simulink model "Quadcopter"  (R2024b)
settings: Solver=VariableStepAuto  StartTime=0.0  StopTime=1000  FixedStep=0.0001  RelTol=1e-3
values from neighbouring files (symbols this model uses):
  f = fn{i}    [LandingAnalysis.m]    (also in PerformanceAnalysis.m = @(a) obj.lift_residual(alt,V,M,rho,L_target,a,throttle); TakeoffAnalysis.m)
undefined symbols (not defined in the file or in its folder): Earth, WGS84
libraries: slpidlib x5, simulink_extras x2, aerolibfltsims x2, instrumentlib x2, shared6dof x1, vrlib x1, aerolibtransform2 x1, aerolibanimutils x1
settings Model: Creator=naman  LastModifiedBy=naman

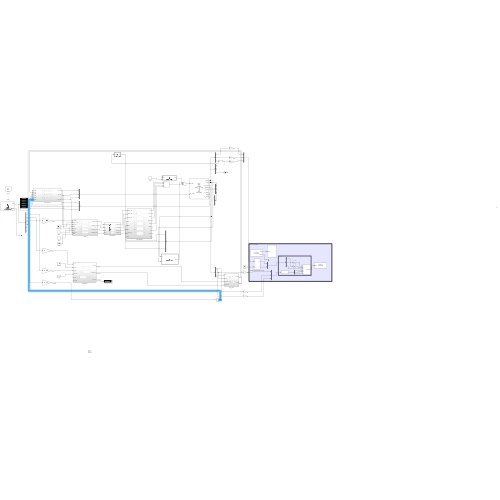
[thumbnail: Simulink's stored preview of the top-level diagram]
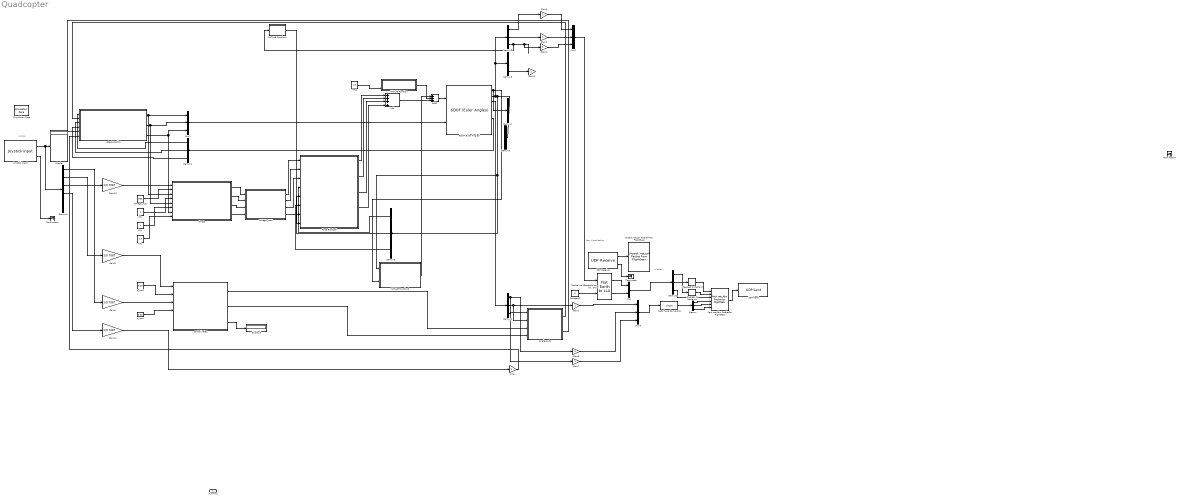
== system Quadcopter ==
  note: proiler
  note: Inertial
  note: New Visualization
  6DOF (Euler Angles) : shared6dof/6DOF (Euler Angles)  units=Metric (MKS)  mtype=Fixed  rep=Euler Angles  xme_0=[0;0;0]  Vm_0=[0;0;0]  eul_0=[0;0;0]  pm_0=[0;0;0]  mass_0=1.5  mass_e=0.5  mass_f=2.0  inertia=[0.06 0 0;0 0.06 0;0 0 0.10]  inertia_e=eye(3)  inertia_f=2*eye(3)  k_quat=1.0  vre_flag=on  abi_flag=off  aMode=0  xme_statename=''  Vm_statename=''  eul_statename=''  quat_statename=''  pm_statename=''  mass_statename=''
  Add : Sum  Inputs=++++
  Add2 : Sum  Inputs=+++
  Constant2 : Constant  Value=0
  Data Type Conversion : DataTypeConversion  OutDataTypeStr=single  SaturateOnIntegerOverflow=off  RndMeth=Floor
  Degrees to Radians : simulink_extras/Transformations/Degrees to Radians
  Degrees to Radians1 : simulink_extras/Transformations/Degrees to Radians
  Demux{,1..8} (9 alike) : Demux  Outputs=3
  Demux9 : Demux  Outputs=6
  Display : Display
  Display1 : Display
  Force Blockset : Subsystem
  Gain{1..4,6..7} (6 alike) : Gain
  Gain{8..11} (4 alike) : Gain  Gain=1/0.7087
  Gain5 : Gain  Gain=-1
  Joystick Input : vrlib/Joystick Input  joyid=1  adjustports=on  forcefeed=off
  MATLAB Function : MATLAB Function  TreatAsAtomicUnit=on
  MATLAB Function1 : MATLAB Function  TreatAsAtomicUnit=on
  MATLAB Function3 : MATLAB Function  TreatAsAtomicUnit=on
  Mux : Mux  Inputs=2
  Mux1 : Mux  Inputs=3
  Mux2 : Mux  Inputs=3
  Mux3 : Mux  Inputs=3
  Omega_max : Constant  Value=950
  Omega_rotor : Subsystem
  Omga : Subsystem
  Pack net_fdm Packet for FlightGear : aerolibfltsims/Pack net_fdm Packet for FlightGear  FlightGearVersion=v2019.1  ShowPositionAttitudeInputs=on  ShowVelocityAccelerationInputs=off  ShowControlSurfacePositionInputs=off  ShowEngineFuelInputs=off  ShowLandingGearInputs=off  ShowEnvironmentInputs=off  SampleTime=-1  packetVersion=24
  "Position to [Geodetic lat, lon, alti]" : aerolibtransform2/Flat Earth to LLA  units=Metric (MKS)  ptype=Earth (WGS84)  F=1/298.257223563  R=6378137  refPosPort=off  LL0=[37.210265015306916, -80.41446644179189]  psi=0
  Simulation Pace : aerolibanimutils/Simulation Pace  SimulationPace=1  SleepMode=Auto  OutputPaceError=off  SampleTime=1/30
  Terminator : Terminator
  Terminator1 : Terminator
  Terminator4 : Terminator
  UDP Receive : instrumentlib/UDP Receive  LocalAddress=127.0.0.1  LocalPort=50001  EnablePortSharing=off  Host=localhost  Port=65343  GetLatestData=on  DataSize=[ 1, 744 ]  DataType=uint8  ASCIIFormatting=%f,  Terminator=LF  CustomTerminator=10  ByteOrder=little-endian  EnableBlockingMode=off  Timeout=10  SampleTime=0.2  SimulateUsing=Interpreted execution
  UDP Send : instrumentlib/UDP Send  Host=localhost  Port=50000  LocalAddress=127.0.0.1  LocalPort=-1  EnablePortSharing=on  OutputDatagramPacketSize=4096  ByteOrder=big-endian  EnableBlockingMode=on  SimulateUsing=Interpreted execution
  Unpack net_ctrl Packet from FlightGear : aerolibfltsims/Unpack net_ctrl Packet from FlightGear  FlightGearVersion=v2019.1  ShowControlSurfacePositionOutputs=off  ShowEngineFuelOutputs=off  ShowLandingGearOutputs=off  ShowAvionicOutputs=off  ShowEnvironmentOutputs=off  SampleTime=-1  packetVersion=27
  angle_auto : Subsystem
  controll rates : Subsystem
  kMx : Constant  Value=4
  kMy : Constant  Value=4
  kMz : Constant  Value=1.5
  mass : Constant  Value=1.5
  p_max : Constant  Value=0.35
  q_max : Constant  Value=0.35
  r_max : Gain
  rate_Autopilot : Subsystem
  dummy2 : Outport
  wires:
  Demux/2 -> Pack net_fdm Packet for FlightGear/5
  Gain10/1 -> Omga/1(u_throttle)  "throttle"
  rate_Autopilot/1(Mx_cmd) -> Omga/3(Mx_cmd), Mux2/1
  kMz/1 -> Omga/8(kMz)
  Demux1/1 -> Degrees to Radians1/1
  Gain2/1 -> Mux1/2  "theta"
  Degrees to Radians1/1 -> Pack net_fdm Packet for FlightGear/2
  Degrees to Radians/1 -> Pack net_fdm Packet for FlightGear/1
  Demux/1 -> Pack net_fdm Packet for FlightGear/4
  controll rates/1(phi_cmd) -> angle_auto/3(phi_cmd)  "phi_cmd"
  Demux1/3 -> Pack net_fdm Packet for FlightGear/3
  Demux1/2 -> Degrees to Radians/1
  Data Type Conversion/1 -> Demux/1
  Omega_rotor/1(omega_FR) -> Force Blockset/1(Omega_FR)
  Demux/3 -> Pack net_fdm Packet for FlightGear/6
  Demux8/3 -> Force Blockset/6(psi)
  mass/1 -> MATLAB Function/3(m)
  UDP Receive/1 -> Unpack net_ctrl Packet from FlightGear/1
  rate_Autopilot/3(Mz_cmd) -> Omga/7(Mz_cmd), Mux2/3
  Demux9/2 -> Gain9/1  "roll"
  UDP Receive/2 -> Terminator/1
  Demux8/2 -> Force Blockset/5(theta)
  "Position to [Geodetic lat, lon, alti]"/1 -> Mux/1
  "Position to [Geodetic lat, lon, alti]"/2 -> Mux/2
  controll rates/3(psi_cmd) -> Display1/1  "psi_cmd"
  Omega_rotor/3(omega_RL) -> Force Blockset/3(Omega_RL)
  Joystick Input/1 -> Display/1, Demux9/1
  Joystick Input/2 -> Terminator1/1
  Demux9/1 -> Gain8/1
  q_max/1 -> controll rates/4(theta_max)
  Demux9/3 -> Gain10/1  "throttle"
  Demux8/1 -> Force Blockset/4(phi)
  Demux9/4 -> Gain11/1  "YAW"
  Force Blockset/5(Rrad) -> Add/3
  rate_Autopilot/2(My_cmd) -> Omga/5(My_cmd), Mux2/2
  Demux4/2 -> rate_Autopilot/3(q_6dof)
  Omega_max/1 -> Omga/2(Omega_max)
  Demux4/1 -> rate_Autopilot/1(p_6dof)
  kMx/1 -> Omga/4(kMx)
  kMy/1 -> Omga/6(kMy)
  Gain9/1 -> controll rates/1(u_roll)  "roll"
  p_max/1 -> controll rates/2(phi_max)
  Gain8/1 -> controll rates/3(u_pitch)  "pitch"
  Add/1 -> Add2/3
  Gain11/1 -> r_max/1  "u_yawYAW"
  Force Blockset/1(Front) -> Add/1
  MATLAB Function1/1(rho) -> Force Blockset/8(rho)
  Demux4/3 -> rate_Autopilot/4(r_6dof)
  Mux2/1 -> 6DOF (Euler Angles)/2
  Omga/1(Omega_base) -> Omega_rotor/1(Omega_base)
  Omga/2(dOmega_roll) -> Omega_rotor/2(dOr)
  Omga/3(dOmega_pitch) -> Omega_rotor/3(dOp)
  Omega_rotor/2(omega_RR) -> Force Blockset/2(Omega_RR)
  Omga/4(dOmega_yaw) -> Omega_rotor/4(dOy)
  controll rates/2(theta_cmd) -> angle_auto/4(theat_cmd)  "theta_cmd"
  Omega_rotor/4(omega_FL) -> Force Blockset/7(Omega_FL)
  Force Blockset/3(Right) -> Add/2
  Force Blockset/7(left) -> Add/4
  MATLAB Function/1(Fg_b) -> Add2/2
  MATLAB Function3/1(Fgnd_n) -> Add2/1
  Add2/1 -> 6DOF (Euler Angles)/1
  6DOF (Euler Angles)/1 -> Demux7/1, MATLAB Function3/2(Ve)
  6DOF (Euler Angles)/2 -> Demux8/1, MATLAB Function3/1(Xe), Demux6/1, Demux5/1, Demux2/1
  6DOF (Euler Angles)/3 -> Demux3/1
  6DOF (Euler Angles)/6 -> Demux4/1
  Demux2/1 -> Gain3/1
  Demux2/2 -> Gain2/1
  Demux2/3 -> Gain4/1, MATLAB Function1/1(Z_ned)  "z axis"
  Demux5/3 -> Gain5/1
  Demux3/1 -> Gain6/1, angle_auto/1(phi)  "phi"
  Demux3/2 -> Gain1/1, angle_auto/2(theta)  "theta"
  Demux3/3 -> Gain7/1  "psi"
  Gain3/1 -> Mux1/1  "phi"
  Gain4/1 -> Mux1/3  "psi"
  angle_auto/1(p_cmd) -> rate_Autopilot/2(p_cmd)  "p_cmd"
  angle_auto/2(q_cmd) -> rate_Autopilot/5(q_cmd)  "q_cmd"
  Pack net_fdm Packet for FlightGear/1 -> UDP Send/1
  Mux/1 -> Demux1/1
  Mux3/1 -> Data Type Conversion/1
  Mux1/1 -> "Position to [Geodetic lat, lon, alti]"/1
  Constant2/1 -> "Position to [Geodetic lat, lon, alti]"/2
  Gain1/1 -> Mux3/1  "theta"
  Gain6/1 -> Mux3/2  "phi"
  Gain7/1 -> Mux3/3  "psi"
  r_max/1 -> rate_Autopilot/6(r_cmd)  "r_cmd"

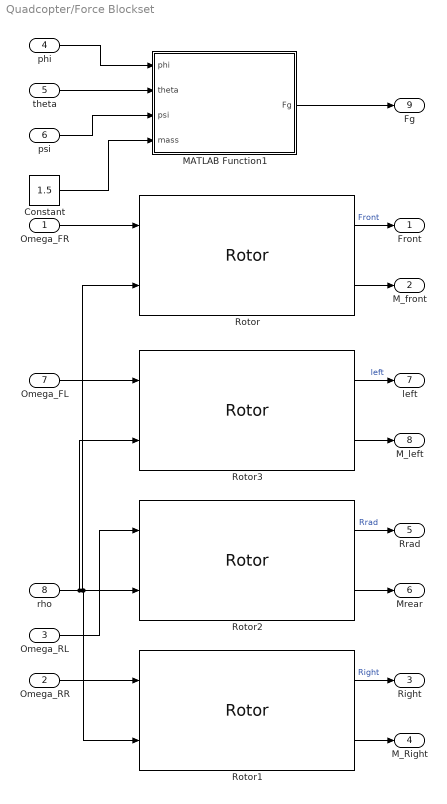
== system Quadcopter/Force Blockset ==
  Omega_FR : Inport
  Omega_RR : Inport  Port=2
  Omega_RL : Inport  Port=3
  phi : Inport  Port=4
  theta : Inport  Port=5
  psi : Inport  Port=6
  Omega_FL : Inport  Port=7
  rho : Inport  Port=8
  Constant : Constant  Value=1.5
  MATLAB Function1 : MATLAB Function  TreatAsAtomicUnit=on
  Rotor{,1..3} (4 alike) : Rotor  radius=0.127
  Front : Outport
  M_front : Outport  Port=2
  Right : Outport  Port=3
  M_Right : Outport  Port=4
  Rrad : Outport  Port=5
  Mrear : Outport  Port=6
  left : Outport  Port=7
  M_left : Outport  Port=8
  Fg : Outport  Port=9
  wires:
  phi/1 -> MATLAB Function1/1(phi)
  Omega_FL/1 -> Rotor3/1
  Omega_RL/1 -> Rotor2/1
  rho/1 -> Rotor1/2, Rotor2/2, Rotor/2, Rotor3/2
  theta/1 -> MATLAB Function1/2(theta)
  Omega_FR/1 -> Rotor/1
  Omega_RR/1 -> Rotor1/1
  psi/1 -> MATLAB Function1/3(psi)
  Constant/1 -> MATLAB Function1/4(mass)
  MATLAB Function1/1(Fg) -> Fg/1
  Rotor3/2 -> M_left/1
  Rotor/1 -> Front/1  "Front"
  Rotor/2 -> M_front/1
  Rotor3/1 -> left/1  "left"
  Rotor2/1 -> Rrad/1  "Rrad"
  Rotor2/2 -> Mrear/1
  Rotor1/1 -> Right/1  "Right"
  Rotor1/2 -> M_Right/1

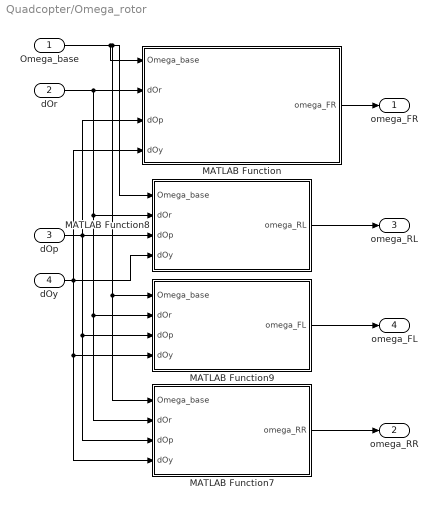
== system Quadcopter/Omega_rotor ==
  Omega_base : Inport
  dOr : Inport  Port=2
  dOp : Inport  Port=3
  dOy : Inport  Port=4
  MATLAB Function : MATLAB Function  TreatAsAtomicUnit=on
  MATLAB Function7 : MATLAB Function  TreatAsAtomicUnit=on
  MATLAB Function8 : MATLAB Function  TreatAsAtomicUnit=on
  MATLAB Function9 : MATLAB Function  TreatAsAtomicUnit=on
  omega_FR : Outport
  omega_RR : Outport  Port=2
  omega_RL : Outport  Port=3
  omega_FL : Outport  Port=4
  wires:
  MATLAB Function7/1(omega_RR) -> omega_RR/1
  MATLAB Function/1(omega_FR) -> omega_FR/1
  Omega_base/1 -> MATLAB Function9/1(Omega_base), MATLAB Function7/1(Omega_base), MATLAB Function8/1(Omega_base), MATLAB Function/1(Omega_base)
  dOy/1 -> MATLAB Function9/4(dOy), MATLAB Function7/4(dOy), MATLAB Function8/4(dOy), MATLAB Function/4(dOy)
  dOp/1 -> MATLAB Function9/3(dOp), MATLAB Function7/3(dOp), MATLAB Function8/3(dOp), MATLAB Function/3(dOp)
  dOr/1 -> MATLAB Function9/2(dOr), MATLAB Function7/2(dOr), MATLAB Function8/2(dOr), MATLAB Function/2(dOr)
  MATLAB Function8/1(omega_RL) -> omega_RL/1
  MATLAB Function9/1(omega_FL) -> omega_FL/1

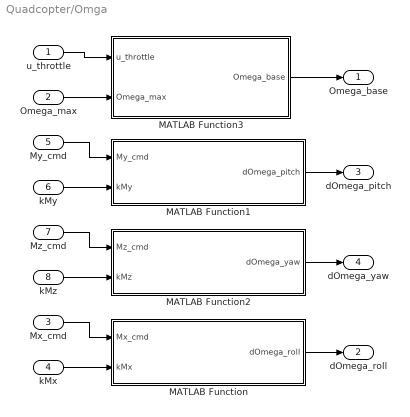
== system Quadcopter/Omga ==
  u_throttle : Inport
  Omega_max : Inport  Port=2
  Mx_cmd : Inport  Port=3
  kMx : Inport  Port=4
  My_cmd : Inport  Port=5
  kMy : Inport  Port=6
  Mz_cmd : Inport  Port=7
  kMz : Inport  Port=8
  MATLAB Function : MATLAB Function  TreatAsAtomicUnit=on
  MATLAB Function1 : MATLAB Function  TreatAsAtomicUnit=on
  MATLAB Function2 : MATLAB Function  TreatAsAtomicUnit=on
  MATLAB Function3 : MATLAB Function  TreatAsAtomicUnit=on
  Omega_base : Outport
  dOmega_roll : Outport  Port=2
  dOmega_pitch : Outport  Port=3
  dOmega_yaw : Outport  Port=4
  wires:
  Mx_cmd/1 -> MATLAB Function/1(Mx_cmd)
  Mz_cmd/1 -> MATLAB Function2/1(Mz_cmd)
  My_cmd/1 -> MATLAB Function1/1(My_cmd)
  u_throttle/1 -> MATLAB Function3/1(u_throttle)
  kMx/1 -> MATLAB Function/2(kMx)
  kMz/1 -> MATLAB Function2/2(kMz)
  kMy/1 -> MATLAB Function1/2(kMy)
  Omega_max/1 -> MATLAB Function3/2(Omega_max)
  MATLAB Function3/1(Omega_base) -> Omega_base/1
  MATLAB Function1/1(dOmega_pitch) -> dOmega_pitch/1
  MATLAB Function2/1(dOmega_yaw) -> dOmega_yaw/1
  MATLAB Function/1(dOmega_roll) -> dOmega_roll/1

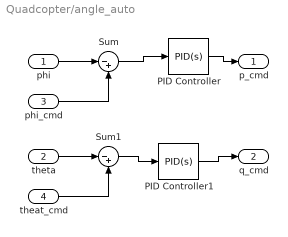
== system Quadcopter/angle_auto ==
  phi : Inport
  theta : Inport  Port=2
  phi_cmd : Inport  Port=3
  theat_cmd : Inport  Port=4
  PID Controller : slpidlib/PID Controller  Controller=PID  Form=Parallel  TimeDomain=Continuous-time  UseExternalTs=off  SampleTime=-1  IntegratorMethod=Forward Euler  FilterMethod=Forward Euler  ControllerParametersSource=internal  P=2.14402423687846  I=0.491971339877455  UseKiTs=off  D=2.26060343958591  UseExternalDerivativeSource=off  N=243.403008728026  UseFilter=on  TunerSelectOption=Transfer Function Based (PID Tuner App)  InitialConditionSource=internal  InitialConditionForIntegrator=0  InitialConditionForFilter=0  DifferentiatorICPrevScaledInput=0  ExternalReset=none  TrackingMode=off  Kt=1  LimitOutput=off  SatLimitsSource=internal  UpperSaturationLimit=inf  LowerSaturationLimit=-inf  LinearizeAsGain=on  AntiWindupMode=none  Kb=1  LimitIntegrator=off  UpperIntegratorSaturationLimit=inf  LowerIntegratorSaturationLimit=-inf  POutMin=[]  POutMax=[]  IOutMin=[]  IOutMax=[]  DOutMin=[]  DOutMax=[]  NOutMin=[]  NOutMax=[]  SumOutMin=[]  SumOutMax=[]  SaturationOutMin=[]  SaturationOutMax=[]  PParamMin=[]  PParamMax=[]  IParamMin=[]  IParamMax=[]  DParamMin=[]  DParamMax=[]  NParamMin=[]  NParamMax=[]  KbParamMin=[]  KbParamMax=[]  KtParamMin=[]  KtParamMax=[]  KbOutMin=[]  KbOutMax=[]  KtOutMin=[]  KtOutMax=[]  IntegratorOutMin=[]  IntegratorOutMax=[]  FilterOutMin=[]  FilterOutMax=[]  SumI1OutMin=[]  SumI1OutMax=[]  SumI2OutMin=[]  SumI2OutMax=[]  SumI3OutMin=[]  SumI3OutMax=[]  SumI4OutMin=[]  SumI4OutMax=[]  SumDOutMin=[]  SumDOutMax=[]  DifferentiatorOutMin=[]  DifferentiatorOutMax=[]  FilterDiffOutCoefMin=[]  FilterDiffOutCoefMax=[]  ReciprocalOutMin=[]  ReciprocalOutMax=[]  SumDenOutMin=[]  SumDenOutMax=[]  SumNumOutMin=[]  SumNumOutMax=[]  DivideOutMin=[]  DivideOutMax=[]  UdiffTsProdOutMin=[]  UdiffTsProdOutMax=[]  NTsProdOutMin=[]  NTsProdOutMax=[]  UintegralTsProdOutMin=[]  UintegralTsProdOutMax=[]  UngainTsProdOutMin=[]  UngainTsProdOutMax=[]  ClampingZeroOutDataTypeStr=Inherit: Inherit via back propagation  ClampingZeroOutMin=[]  ClampingZeroOutMax=[]  FilterDenConstantOutDataTypeStr=Inherit: Inherit via back propagation  FilterDenConstantOutMin=[]  FilterDenConstantOutMax=[]  PCopyOutDataTypeStr=Inherit: Inherit via back propagation  PCopyOutMin=[]  PCopyOutMax=[]  NCopyOutDataTypeStr=Inherit: Inherit via back propagation  NCopyOutMin=[]  NCopyOutMax=[]  IntegratorContinuousStateAttributes=''  IntegratorStateMustResolveToSignalObject=off  IntegratorRTWStateStorageClass=Auto  FilterContinuousStateAttributes=''  FilterStateMustResolveToSignalObject=off  FilterRTWStateStorageClass=Auto  ParallelPVariant=InternalParameters  IdealPVariant=Disabled  IVariant=InternalParameters  DVariant=InternalParameters  IntegratorVariant=Continuous  SatVariant=Disabled  AWVariant=Passthrough  PCopyVariant=Disabled  TRVariant=Disabled  FdbkBlocksVariant=Forward  IdealPFdbkVariant=Disabled  SatFdbkVariant=Disabled  DerivativeFilterVariant=ContFilter  NVariant=InternalParameters  NCopyVariant=Disabled  FilterICVariant=InternalICsFilter  IntegratorICVariant=InternalICs  ExternalResetVariant=Disabled  TRSumVariant=Passthrough  SumFdbkVariant=Disabled  SumVariant=Sum_PID  TsampFilterVariant=InternalTs  TsampNgainVariant=Passthrough  TsampIntegralVariant=Disabled_SignalSpec  ExternalSaturationOutDataTypeStr=Inherit: Same as second input  DerivativeSourceVariant=ErrorSignal  PreIntVariant=InternalPreInt
  PID Controller1 : slpidlib/PID Controller  Controller=PID  Form=Parallel  TimeDomain=Continuous-time  UseExternalTs=off  SampleTime=-1  IntegratorMethod=Forward Euler  FilterMethod=Forward Euler  ControllerParametersSource=internal  P=2.4550641196179  I=0.68497255926485  UseKiTs=off  D=2.17640567319301  UseExternalDerivativeSource=off  N=317.566046248677  UseFilter=on  TunerSelectOption=Transfer Function Based (PID Tuner App)  InitialConditionSource=internal  InitialConditionForIntegrator=0  InitialConditionForFilter=0  DifferentiatorICPrevScaledInput=0  ExternalReset=none  TrackingMode=off  Kt=1  LimitOutput=off  SatLimitsSource=internal  UpperSaturationLimit=inf  LowerSaturationLimit=-inf  LinearizeAsGain=on  AntiWindupMode=none  Kb=1  LimitIntegrator=off  UpperIntegratorSaturationLimit=inf  LowerIntegratorSaturationLimit=-inf  POutMin=[]  POutMax=[]  IOutMin=[]  IOutMax=[]  DOutMin=[]  DOutMax=[]  NOutMin=[]  NOutMax=[]  SumOutMin=[]  SumOutMax=[]  SaturationOutMin=[]  SaturationOutMax=[]  PParamMin=[]  PParamMax=[]  IParamMin=[]  IParamMax=[]  DParamMin=[]  DParamMax=[]  NParamMin=[]  NParamMax=[]  KbParamMin=[]  KbParamMax=[]  KtParamMin=[]  KtParamMax=[]  KbOutMin=[]  KbOutMax=[]  KtOutMin=[]  KtOutMax=[]  IntegratorOutMin=[]  IntegratorOutMax=[]  FilterOutMin=[]  FilterOutMax=[]  SumI1OutMin=[]  SumI1OutMax=[]  SumI2OutMin=[]  SumI2OutMax=[]  SumI3OutMin=[]  SumI3OutMax=[]  SumI4OutMin=[]  SumI4OutMax=[]  SumDOutMin=[]  SumDOutMax=[]  DifferentiatorOutMin=[]  DifferentiatorOutMax=[]  FilterDiffOutCoefMin=[]  FilterDiffOutCoefMax=[]  ReciprocalOutMin=[]  ReciprocalOutMax=[]  SumDenOutMin=[]  SumDenOutMax=[]  SumNumOutMin=[]  SumNumOutMax=[]  DivideOutMin=[]  DivideOutMax=[]  UdiffTsProdOutMin=[]  UdiffTsProdOutMax=[]  NTsProdOutMin=[]  NTsProdOutMax=[]  UintegralTsProdOutMin=[]  UintegralTsProdOutMax=[]  UngainTsProdOutMin=[]  UngainTsProdOutMax=[]  ClampingZeroOutDataTypeStr=Inherit: Inherit via back propagation  ClampingZeroOutMin=[]  ClampingZeroOutMax=[]  FilterDenConstantOutDataTypeStr=Inherit: Inherit via back propagation  FilterDenConstantOutMin=[]  FilterDenConstantOutMax=[]  PCopyOutDataTypeStr=Inherit: Inherit via back propagation  PCopyOutMin=[]  PCopyOutMax=[]  NCopyOutDataTypeStr=Inherit: Inherit via back propagation  NCopyOutMin=[]  NCopyOutMax=[]  IntegratorContinuousStateAttributes=''  IntegratorStateMustResolveToSignalObject=off  IntegratorRTWStateStorageClass=Auto  FilterContinuousStateAttributes=''  FilterStateMustResolveToSignalObject=off  FilterRTWStateStorageClass=Auto  ParallelPVariant=InternalParameters  IdealPVariant=Disabled  IVariant=InternalParameters  DVariant=InternalParameters  IntegratorVariant=Continuous  SatVariant=Disabled  AWVariant=Passthrough  PCopyVariant=Disabled  TRVariant=Disabled  FdbkBlocksVariant=Forward  IdealPFdbkVariant=Disabled  SatFdbkVariant=Disabled  DerivativeFilterVariant=ContFilter  NVariant=InternalParameters  NCopyVariant=Disabled  FilterICVariant=InternalICsFilter  IntegratorICVariant=InternalICs  ExternalResetVariant=Disabled  TRSumVariant=Passthrough  SumFdbkVariant=Disabled  SumVariant=Sum_PID  TsampFilterVariant=InternalTs  TsampNgainVariant=Passthrough  TsampIntegralVariant=Disabled_SignalSpec  ExternalSaturationOutDataTypeStr=Inherit: Same as second input  DerivativeSourceVariant=ErrorSignal  PreIntVariant=InternalPreInt
  Sum : Sum  Inputs=|-+
  Sum1 : Sum  Inputs=|-+
  p_cmd : Outport
  q_cmd : Outport  Port=2
  wires:
  phi/1 -> Sum/1
  phi_cmd/1 -> Sum/2
  Sum/1 -> PID Controller/1
  PID Controller/1 -> p_cmd/1
  PID Controller1/1 -> q_cmd/1
  theat_cmd/1 -> Sum1/2
  theta/1 -> Sum1/1
  Sum1/1 -> PID Controller1/1

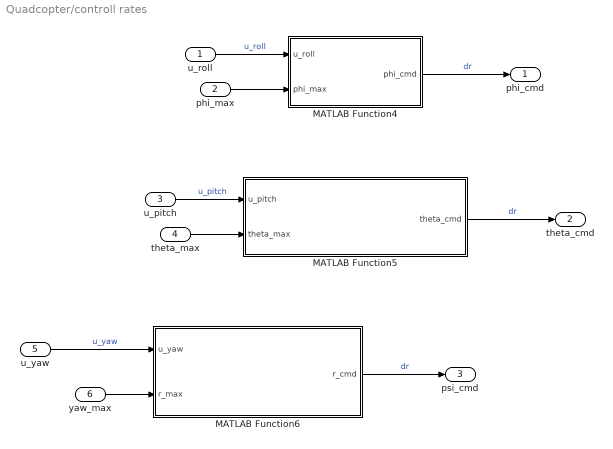
== system Quadcopter/controll rates ==
  u_roll : Inport
  phi_max : Inport  Port=2
  u_pitch : Inport  Port=3
  theta_max : Inport  Port=4
  u_yaw : Inport  Port=5
  yaw_max : Inport  Port=6
  MATLAB Function4 : MATLAB Function  TreatAsAtomicUnit=on
  MATLAB Function5 : MATLAB Function  TreatAsAtomicUnit=on
  MATLAB Function6 : MATLAB Function  TreatAsAtomicUnit=on
  phi_cmd : Outport
  theta_cmd : Outport  Port=2
  psi_cmd : Outport  Port=3
  wires:
  phi_max/1 -> MATLAB Function4/2(phi_max)
  u_roll/1 -> MATLAB Function4/1(u_roll)  "u_roll"
  u_pitch/1 -> MATLAB Function5/1(u_pitch)  "u_pitch"
  theta_max/1 -> MATLAB Function5/2(theta_max)
  u_yaw/1 -> MATLAB Function6/1(u_yaw)  "u_yaw"
  yaw_max/1 -> MATLAB Function6/2(r_max)
  MATLAB Function4/1(phi_cmd) -> phi_cmd/1  "dr"
  MATLAB Function5/1(theta_cmd) -> theta_cmd/1  "dr"
  MATLAB Function6/1(r_cmd) -> psi_cmd/1  "dr"

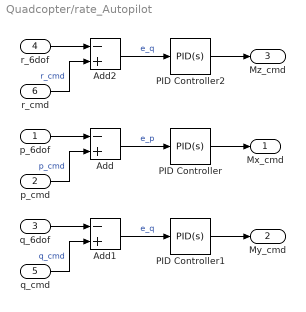
== system Quadcopter/rate_Autopilot ==
  p_6dof : Inport
  p_cmd : Inport  Port=2
  q_6dof : Inport  Port=3
  r_6dof : Inport  Port=4
  q_cmd : Inport  Port=5
  r_cmd : Inport  Port=6
  Add : Sum  Inputs=-+
  Add1 : Sum  Inputs=-+
  Add2 : Sum  Inputs=-+
  PID Controller : slpidlib/PID Controller  Controller=PID  Form=Parallel  TimeDomain=Continuous-time  UseExternalTs=off  SampleTime=-1  IntegratorMethod=Forward Euler  FilterMethod=Forward Euler  ControllerParametersSource=internal  P=0.0616583905012417  I=0.0117941610160119  UseKiTs=off  D=-0.0129936698510517  UseExternalDerivativeSource=off  N=1.72044274974478  UseFilter=on  TunerSelectOption=Transfer Function Based (PID Tuner App)  InitialConditionSource=internal  InitialConditionForIntegrator=0  InitialConditionForFilter=0  DifferentiatorICPrevScaledInput=0  ExternalReset=none  TrackingMode=off  Kt=1  LimitOutput=off  SatLimitsSource=internal  UpperSaturationLimit=inf  LowerSaturationLimit=-inf  LinearizeAsGain=on  AntiWindupMode=none  Kb=1  LimitIntegrator=off  UpperIntegratorSaturationLimit=inf  LowerIntegratorSaturationLimit=-inf  POutMin=[]  POutMax=[]  IOutMin=[]  IOutMax=[]  DOutMin=[]  DOutMax=[]  NOutMin=[]  NOutMax=[]  SumOutMin=[]  SumOutMax=[]  SaturationOutMin=[]  SaturationOutMax=[]  PParamMin=[]  PParamMax=[]  IParamMin=[]  IParamMax=[]  DParamMin=[]  DParamMax=[]  NParamMin=[]  NParamMax=[]  KbParamMin=[]  KbParamMax=[]  KtParamMin=[]  KtParamMax=[]  KbOutMin=[]  KbOutMax=[]  KtOutMin=[]  KtOutMax=[]  IntegratorOutMin=[]  IntegratorOutMax=[]  FilterOutMin=[]  FilterOutMax=[]  SumI1OutMin=[]  SumI1OutMax=[]  SumI2OutMin=[]  SumI2OutMax=[]  SumI3OutMin=[]  SumI3OutMax=[]  SumI4OutMin=[]  SumI4OutMax=[]  SumDOutMin=[]  SumDOutMax=[]  DifferentiatorOutMin=[]  DifferentiatorOutMax=[]  FilterDiffOutCoefMin=[]  FilterDiffOutCoefMax=[]  ReciprocalOutMin=[]  ReciprocalOutMax=[]  SumDenOutMin=[]  SumDenOutMax=[]  SumNumOutMin=[]  SumNumOutMax=[]  DivideOutMin=[]  DivideOutMax=[]  UdiffTsProdOutMin=[]  UdiffTsProdOutMax=[]  NTsProdOutMin=[]  NTsProdOutMax=[]  UintegralTsProdOutMin=[]  UintegralTsProdOutMax=[]  UngainTsProdOutMin=[]  UngainTsProdOutMax=[]  ClampingZeroOutDataTypeStr=Inherit: Inherit via back propagation  ClampingZeroOutMin=[]  ClampingZeroOutMax=[]  FilterDenConstantOutDataTypeStr=Inherit: Inherit via back propagation  FilterDenConstantOutMin=[]  FilterDenConstantOutMax=[]  PCopyOutDataTypeStr=Inherit: Inherit via back propagation  PCopyOutMin=[]  PCopyOutMax=[]  NCopyOutDataTypeStr=Inherit: Inherit via back propagation  NCopyOutMin=[]  NCopyOutMax=[]  IntegratorContinuousStateAttributes=''  IntegratorStateMustResolveToSignalObject=off  IntegratorRTWStateStorageClass=Auto  FilterContinuousStateAttributes=''  FilterStateMustResolveToSignalObject=off  FilterRTWStateStorageClass=Auto  ParallelPVariant=InternalParameters  IdealPVariant=Disabled  IVariant=InternalParameters  DVariant=InternalParameters  IntegratorVariant=Continuous  SatVariant=Disabled  AWVariant=Passthrough  PCopyVariant=Disabled  TRVariant=Disabled  FdbkBlocksVariant=Forward  IdealPFdbkVariant=Disabled  SatFdbkVariant=Disabled  DerivativeFilterVariant=ContFilter  NVariant=InternalParameters  NCopyVariant=Disabled  FilterICVariant=InternalICsFilter  IntegratorICVariant=InternalICs  ExternalResetVariant=Disabled  TRSumVariant=Passthrough  SumFdbkVariant=Disabled  SumVariant=Sum_PID  TsampFilterVariant=InternalTs  TsampNgainVariant=Passthrough  TsampIntegralVariant=Disabled_SignalSpec  ExternalSaturationOutDataTypeStr=Inherit: Same as second input  DerivativeSourceVariant=ErrorSignal  PreIntVariant=InternalPreInt
  PID Controller1 : slpidlib/PID Controller  Controller=PID  Form=Parallel  TimeDomain=Continuous-time  UseExternalTs=off  SampleTime=-1  IntegratorMethod=Forward Euler  FilterMethod=Forward Euler  ControllerParametersSource=internal  P=0.101931580790253  I=0.0529903166966982  UseKiTs=off  D=-0.000163696296921277  UseExternalDerivativeSource=off  N=622.687151189941  UseFilter=on  TunerSelectOption=Transfer Function Based (PID Tuner App)  InitialConditionSource=internal  InitialConditionForIntegrator=0  InitialConditionForFilter=0  DifferentiatorICPrevScaledInput=0  ExternalReset=none  TrackingMode=off  Kt=1  LimitOutput=off  SatLimitsSource=internal  UpperSaturationLimit=inf  LowerSaturationLimit=-inf  LinearizeAsGain=on  AntiWindupMode=none  Kb=1  LimitIntegrator=off  UpperIntegratorSaturationLimit=inf  LowerIntegratorSaturationLimit=-inf  POutMin=[]  POutMax=[]  IOutMin=[]  IOutMax=[]  DOutMin=[]  DOutMax=[]  NOutMin=[]  NOutMax=[]  SumOutMin=[]  SumOutMax=[]  SaturationOutMin=[]  SaturationOutMax=[]  PParamMin=[]  PParamMax=[]  IParamMin=[]  IParamMax=[]  DParamMin=[]  DParamMax=[]  NParamMin=[]  NParamMax=[]  KbParamMin=[]  KbParamMax=[]  KtParamMin=[]  KtParamMax=[]  KbOutMin=[]  KbOutMax=[]  KtOutMin=[]  KtOutMax=[]  IntegratorOutMin=[]  IntegratorOutMax=[]  FilterOutMin=[]  FilterOutMax=[]  SumI1OutMin=[]  SumI1OutMax=[]  SumI2OutMin=[]  SumI2OutMax=[]  SumI3OutMin=[]  SumI3OutMax=[]  SumI4OutMin=[]  SumI4OutMax=[]  SumDOutMin=[]  SumDOutMax=[]  DifferentiatorOutMin=[]  DifferentiatorOutMax=[]  FilterDiffOutCoefMin=[]  FilterDiffOutCoefMax=[]  ReciprocalOutMin=[]  ReciprocalOutMax=[]  SumDenOutMin=[]  SumDenOutMax=[]  SumNumOutMin=[]  SumNumOutMax=[]  DivideOutMin=[]  DivideOutMax=[]  UdiffTsProdOutMin=[]  UdiffTsProdOutMax=[]  NTsProdOutMin=[]  NTsProdOutMax=[]  UintegralTsProdOutMin=[]  UintegralTsProdOutMax=[]  UngainTsProdOutMin=[]  UngainTsProdOutMax=[]  ClampingZeroOutDataTypeStr=Inherit: Inherit via back propagation  ClampingZeroOutMin=[]  ClampingZeroOutMax=[]  FilterDenConstantOutDataTypeStr=Inherit: Inherit via back propagation  FilterDenConstantOutMin=[]  FilterDenConstantOutMax=[]  PCopyOutDataTypeStr=Inherit: Inherit via back propagation  PCopyOutMin=[]  PCopyOutMax=[]  NCopyOutDataTypeStr=Inherit: Inherit via back propagation  NCopyOutMin=[]  NCopyOutMax=[]  IntegratorContinuousStateAttributes=''  IntegratorStateMustResolveToSignalObject=off  IntegratorRTWStateStorageClass=Auto  FilterContinuousStateAttributes=''  FilterStateMustResolveToSignalObject=off  FilterRTWStateStorageClass=Auto  ParallelPVariant=InternalParameters  IdealPVariant=Disabled  IVariant=InternalParameters  DVariant=InternalParameters  IntegratorVariant=Continuous  SatVariant=Disabled  AWVariant=Passthrough  PCopyVariant=Disabled  TRVariant=Disabled  FdbkBlocksVariant=Forward  IdealPFdbkVariant=Disabled  SatFdbkVariant=Disabled  DerivativeFilterVariant=ContFilter  NVariant=InternalParameters  NCopyVariant=Disabled  FilterICVariant=InternalICsFilter  IntegratorICVariant=InternalICs  ExternalResetVariant=Disabled  TRSumVariant=Passthrough  SumFdbkVariant=Disabled  SumVariant=Sum_PID  TsampFilterVariant=InternalTs  TsampNgainVariant=Passthrough  TsampIntegralVariant=Disabled_SignalSpec  ExternalSaturationOutDataTypeStr=Inherit: Same as second input  DerivativeSourceVariant=ErrorSignal  PreIntVariant=InternalPreInt
  PID Controller2 : slpidlib/PID Controller  Controller=PID  Form=Parallel  TimeDomain=Continuous-time  UseExternalTs=off  SampleTime=-1  IntegratorMethod=Forward Euler  FilterMethod=Forward Euler  ControllerParametersSource=internal  P=0.102763984168736  I=0.0196569350266865  UseKiTs=off  D=-0.0216561164184195  UseExternalDerivativeSource=off  N=1.72044274974478  UseFilter=on  TunerSelectOption=Transfer Function Based (PID Tuner App)  InitialConditionSource=internal  InitialConditionForIntegrator=0  InitialConditionForFilter=0  DifferentiatorICPrevScaledInput=0  ExternalReset=none  TrackingMode=off  Kt=1  LimitOutput=off  SatLimitsSource=internal  UpperSaturationLimit=inf  LowerSaturationLimit=-inf  LinearizeAsGain=on  AntiWindupMode=none  Kb=1  LimitIntegrator=off  UpperIntegratorSaturationLimit=inf  LowerIntegratorSaturationLimit=-inf  POutMin=[]  POutMax=[]  IOutMin=[]  IOutMax=[]  DOutMin=[]  DOutMax=[]  NOutMin=[]  NOutMax=[]  SumOutMin=[]  SumOutMax=[]  SaturationOutMin=[]  SaturationOutMax=[]  PParamMin=[]  PParamMax=[]  IParamMin=[]  IParamMax=[]  DParamMin=[]  DParamMax=[]  NParamMin=[]  NParamMax=[]  KbParamMin=[]  KbParamMax=[]  KtParamMin=[]  KtParamMax=[]  KbOutMin=[]  KbOutMax=[]  KtOutMin=[]  KtOutMax=[]  IntegratorOutMin=[]  IntegratorOutMax=[]  FilterOutMin=[]  FilterOutMax=[]  SumI1OutMin=[]  SumI1OutMax=[]  SumI2OutMin=[]  SumI2OutMax=[]  SumI3OutMin=[]  SumI3OutMax=[]  SumI4OutMin=[]  SumI4OutMax=[]  SumDOutMin=[]  SumDOutMax=[]  DifferentiatorOutMin=[]  DifferentiatorOutMax=[]  FilterDiffOutCoefMin=[]  FilterDiffOutCoefMax=[]  ReciprocalOutMin=[]  ReciprocalOutMax=[]  SumDenOutMin=[]  SumDenOutMax=[]  SumNumOutMin=[]  SumNumOutMax=[]  DivideOutMin=[]  DivideOutMax=[]  UdiffTsProdOutMin=[]  UdiffTsProdOutMax=[]  NTsProdOutMin=[]  NTsProdOutMax=[]  UintegralTsProdOutMin=[]  UintegralTsProdOutMax=[]  UngainTsProdOutMin=[]  UngainTsProdOutMax=[]  ClampingZeroOutDataTypeStr=Inherit: Inherit via back propagation  ClampingZeroOutMin=[]  ClampingZeroOutMax=[]  FilterDenConstantOutDataTypeStr=Inherit: Inherit via back propagation  FilterDenConstantOutMin=[]  FilterDenConstantOutMax=[]  PCopyOutDataTypeStr=Inherit: Inherit via back propagation  PCopyOutMin=[]  PCopyOutMax=[]  NCopyOutDataTypeStr=Inherit: Inherit via back propagation  NCopyOutMin=[]  NCopyOutMax=[]  IntegratorContinuousStateAttributes=''  IntegratorStateMustResolveToSignalObject=off  IntegratorRTWStateStorageClass=Auto  FilterContinuousStateAttributes=''  FilterStateMustResolveToSignalObject=off  FilterRTWStateStorageClass=Auto  ParallelPVariant=InternalParameters  IdealPVariant=Disabled  IVariant=InternalParameters  DVariant=InternalParameters  IntegratorVariant=Continuous  SatVariant=Disabled  AWVariant=Passthrough  PCopyVariant=Disabled  TRVariant=Disabled  FdbkBlocksVariant=Forward  IdealPFdbkVariant=Disabled  SatFdbkVariant=Disabled  DerivativeFilterVariant=ContFilter  NVariant=InternalParameters  NCopyVariant=Disabled  FilterICVariant=InternalICsFilter  IntegratorICVariant=InternalICs  ExternalResetVariant=Disabled  TRSumVariant=Passthrough  SumFdbkVariant=Disabled  SumVariant=Sum_PID  TsampFilterVariant=InternalTs  TsampNgainVariant=Passthrough  TsampIntegralVariant=Disabled_SignalSpec  ExternalSaturationOutDataTypeStr=Inherit: Same as second input  DerivativeSourceVariant=ErrorSignal  PreIntVariant=InternalPreInt
  Mx_cmd : Outport
  My_cmd : Outport  Port=2
  Mz_cmd : Outport  Port=3
  wires:
  r_6dof/1 -> Add2/1
  Add/1 -> PID Controller/1  "e_p"
  Add2/1 -> PID Controller2/1  "e_q"
  p_cmd/1 -> Add/2  "p_cmd"
  r_cmd/1 -> Add2/2  "r_cmd"
  q_cmd/1 -> Add1/2  "q_cmd"
  PID Controller1/1 -> My_cmd/1
  q_6dof/1 -> Add1/1
  p_6dof/1 -> Add/1
  Add1/1 -> PID Controller1/1  "e_q"
  PID Controller2/1 -> Mz_cmd/1
  PID Controller/1 -> Mx_cmd/1

== matlab function Quadcopter/MATLAB Function1 ==
  data: Z_ned input; rho output
function rho = isa_density(Z_ned)
h = -Z_ned; 
T0 = 288.15;
P0 = 101325;
g  = 9.80665;
R  = 287.05;
L  = 0.0065;

if h < 0
    h = 0;
end

if h <= 11000
    T = T0 - L*h;
    P = P0 * (T/T0)^(g/(R*L));
else
    T = 216.65;
    P11 = P0 * ((T0 - L*11000)/T0)^(g/(R*L));
    P = P11 * exp(-g*(h-11000)/(R*T));
end

rho = P/(R*T);

end

== matlab function Quadcopter/Omga/MATLAB Function1 ==
  data: My_cmd input; dOmega_pitch output; kMy input
function dOmega_pitch = My_to_dOmega(My_cmd, kMy)
dOmega_pitch = kMy * My_cmd;
end

== matlab function Quadcopter/Force Blockset/MATLAB Function1 ==
  data: phi input; Fg output; theta input; psi input; mass input
function Fg = gravity_body(phi, theta, psi, mass)

g = 9.81;

cphi = cos(phi);
sphi = sin(phi);
cth  = cos(theta);
sth  = sin(theta);
cpsi = cos(psi);
spsi = sin(psi);

Cbn = [ ...
    cth*cpsi,                      cth*spsi,                     -sth;
    sphi*sth*cpsi - cphi*spsi,     sphi*sth*spsi + cphi*cpsi,    sphi*cth;
    cphi*sth*cpsi + sphi*spsi,     cphi*sth*spsi - sphi*cpsi,    cphi*cth];
Fg_ned = [0; 0; mass*g];
Fg = Cbn * Fg_ned;

end

== matlab function Quadcopter/Omga/MATLAB Function2 ==
  data: Mz_cmd input; dOmega_yaw output; kMz input
function dOmega_yaw = Mz_to_dOmega(Mz_cmd, kMz)
dOmega_yaw = kMz * Mz_cmd;
end

== matlab function Quadcopter/Omga/MATLAB Function3 ==
  data: u_throttle input; Omega_base output; Omega_max input
function Omega_base = throttle_to_Omega_base(u_throttle, Omega_max)

u_throttle = max(min(u_throttle,1),-1);
thr01 = 0.5*(u_throttle + 1);
Omega_base = Omega_max * thr01;

end

== matlab function Quadcopter/MATLAB Function ==
  data: phi input; theta input; m input; Fg_b output
function Fg_b = gravity_body(phi, theta, m)
g = 9.81;

Fg_b = m*g * [ ...
    -sin(theta);
     sin(phi)*cos(theta);
     cos(phi)*cos(theta)];
end

== matlab function Quadcopter/Omega_rotor/MATLAB Function ==
  data: Omega_base input; omega_FR output; dOr input; dOp input; dOy input
function omega_FR = motor_FR(Omega_base, dOr, dOp, dOy)
Omega_base = Omega_base(1);
dOr = dOr(1);
dOp = dOp(1);
dOy = dOy(1);
omega_FR = Omega_base - dOr - dOp - dOy;

end

== matlab function Quadcopter/Omga/MATLAB Function ==
  data: Mx_cmd input; dOmega_roll output; kMx input
function dOmega_roll = Mx_to_dOmega(Mx_cmd, kMx)
dOmega_roll = kMx * Mx_cmd;
end

== matlab function Quadcopter/MATLAB Function3 ==
  data: Xe input; Fgnd_n output; Ve input
function Fgnd_n = ground_model(Xe, Ve)
Xe = Xe(:);
Ve = Ve(:);

Z  = Xe(3);   
Vz = Ve(3);    
k = 20000;
c = 2000;
Z_ground = 0;

Fgnd_n = zeros(3,1);

pen = Z - Z_ground;

if pen >= 0
    Fz = -k*pen - c*Vz;   % upward = negative NED z
    Fgnd_n(3) = min(Fz,0);
end
end

== matlab function Quadcopter/controll rates/MATLAB Function4 ==
  data: u_roll input; phi_cmd output; phi_max input
function phi_cmd = uroll_to_phicmd(u_roll, phi_max)
u_roll = max(min(u_roll,1),-1);
phi_cmd = phi_max * u_roll;
end

== matlab function Quadcopter/controll rates/MATLAB Function5 ==
  data: u_pitch input; theta_cmd output; theta_max input
function theta_cmd = upitch_to_qcmd(u_pitch, theta_max)

u_pitch = max(min(u_pitch,1),-1);
theta_cmd = theta_max * u_pitch;

end

== matlab function Quadcopter/controll rates/MATLAB Function6 ==
  data: u_yaw input; r_cmd output; r_max input
function r_cmd = uyaw_to_rcmd(u_yaw, r_max)

u_yaw = max(min(u_yaw,1),-1);
r_cmd = r_max * u_yaw;

end

== matlab function Quadcopter/Omega_rotor/MATLAB Function7 ==
  data: Omega_base input; omega_RR output; dOr input; dOp input; dOy input
function omega_RR = motor_RR(Omega_base, dOr, dOp, dOy)
Omega_base = Omega_base(1);
dOr = dOr(1);
dOp = dOp(1);
dOy = dOy(1);
omega_RR = Omega_base - dOr + dOp + dOy;

end

== matlab function Quadcopter/Omega_rotor/MATLAB Function8 ==
  data: Omega_base input; omega_RL output; dOr input; dOp input; dOy input
function omega_RL = motor_RL(Omega_base, dOr, dOp, dOy)
Omega_base = Omega_base(1);
dOr = dOr(1);
dOp = dOp(1);
dOy = dOy(1);
omega_RL = Omega_base + dOr + dOp - dOy;

end

== matlab function Quadcopter/Omega_rotor/MATLAB Function9 ==
  data: Omega_base input; omega_FL output; dOr input; dOp input; dOy input
function omega_FL = motor_FL(Omega_base, dOr, dOp, dOy)
Omega_base = Omega_base(1);
dOr = dOr(1);
dOp = dOp(1);
dOy = dOy(1);
omega_FL = Omega_base + dOr - dOp + dOy;

end
